simulink model "test_xeng_10_1"  (Simulink 7.2)
settings: Solver=ode45  StartTime=0.0  StopTime=400000  RelTol=1e-3
libraries: xbsIndex_r4 x840, xbsReplacements_r4 x72, casper_library x22, xps_library x3, simulink x1
(part 1 of 9)
settings Model: Creator=Jason Manley  LastModifiedBy=root
settings OptimizationCC: InitFltsAndDblsToZero=on

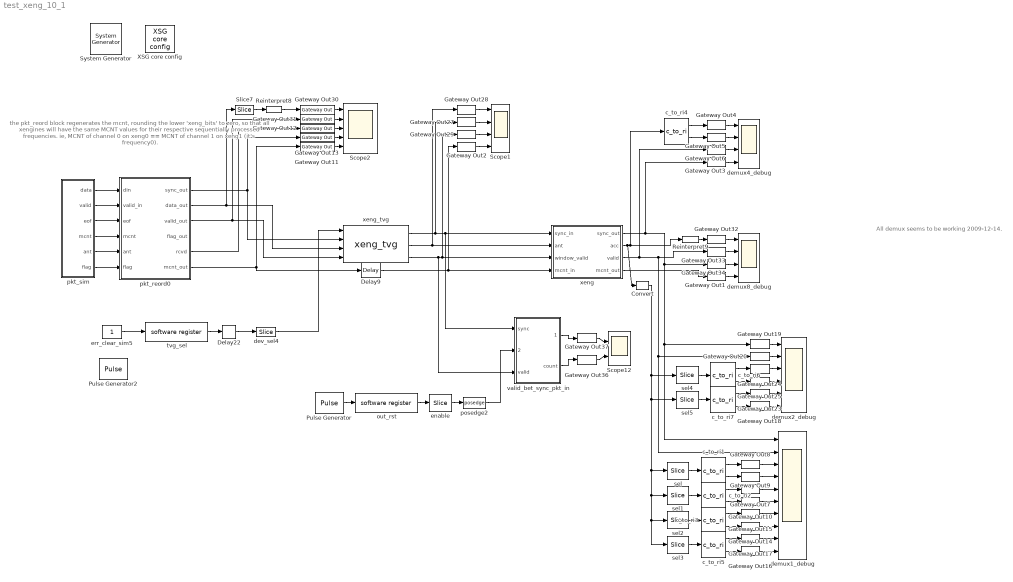
== system test_xeng_10_1 ==
  note: the pkt_reord block regenerates
      | the mcnt, rounding the lower
      | 'xeng_bits' to zero, so that all xengines
      | will have the same MCNT values for their respective
      | sequentially processed frequencies.
      | ie, MCNT of channel 0 on xeng0
      | ==
      | MCNT of channel 1 on xeng1 (it's frequency0).
  note: All demux seems to be working 2009-12-14.
  " System Generator" : xbsIndex_r4/ System Generator  Tag=genX  SystemSampleTime=-1  xilinxfamily=virtex5  part=xc5vlx110t  speed=-1  package=ff1136  synthesis_tool=XST  clock_wrapper=Clock Enables  directory=./test_vacc_pkt_10_1/sysgen  testbench=off  simulink_period=1  sysclk_period=5  dcm_input_clock_period=100  incr_netlist=off  trim_vbits=Everywhere in SubSystem  dbl_ovrd=According to Block Masks  core_generation=According to Block Masks  run_coregen=off  deprecated_control=off  eval_field=0  block_type=sysgen
      settings: block_version=10.1.3
  Convert : xbsIndex_r4/Convert  arith_type=Unsigned  n_bits=128  bin_pt=0  quantization=Truncate  overflow=Wrap  latency=0  dbl_ovrd=off  pipeline=off  block_type=convert
      settings: block_version=10.1.3
  Delay22 : xbsIndex_r4/Delay  en=off  latency=2  dbl_ovrd=off  reg_retiming=off  block_type=delay
      settings: xl_area=[0, 0, 0, 0, 0, 0, 0]
  Delay9 : xbsIndex_r4/Delay  en=off  latency=3  dbl_ovrd=off  reg_retiming=on  block_type=delay
      settings: xl_area=[0, 0, 0, 0, 0, 0, 0]
  Gateway Out{1..10,14..20,23..25,27..29,32..34,36..37} (28 alike) : xbsIndex_r4/Gateway Out  hdl_port=off  timing_constraint=None  locs_specified=off  LOCs={}  block_type=gatewayout
      settings: infoedit="Gateway out block.  Converts Xilinx fixed point inputs into ouputs of type Simulink integer, double, or fixed point.<P><P>Hardware notes:  In hardware these blocks become top level output ports or are discarded, depending on how they are configured."  xl_area=[0, 0, 0, 0, 0, 0, 0]  block_version=10.1.3
  Gateway Out{11..13,30..31} (5 alike) : xbsIndex_r4/Gateway Out  hdl_port=on  timing_constraint=None  locs_specified=off  LOCs={}  block_type=gatewayout
      settings: infoedit="Gateway out block.  Converts Xilinx fixed point inputs into ouputs of type Simulink integer, double, or fixed point.<P><P>Hardware notes:  In hardware these blocks become top level output ports or are discarded, depending on how they are configured."  xl_area=[0, 0, 0, 0, 0, 0, 0]  block_version=10.1.3
  Pulse Generator : DiscretePulseGenerator  Period=2^15  PhaseDelay=2^14
  Pulse Generator2 : DiscretePulseGenerator  Period=100000  PhaseDelay=1
  Reinterpret8 : xbsIndex_r4/Reinterpret  force_arith_type=on  arith_type="Signed  (2's comp)"  force_bin_pt=on  bin_pt=3  block_type=reinterpret
      settings: infoedit="Changes signal type without altering the binary representation.   You can changed the signal between signed and unsigned, and relocate the binary point.<P><P>Hardware notes: In hardware this block costs nothing.<P><P>Example:  Suppose the input is 6 bits wide, signed, with 2 fractional bits, and the output is forced to unsigned with 0 fractional bits.  Then an input of -2.0 (1110.00 in binary 2's complement) becomes an output of 56 (111000 in binary)."  block_version=10.1.3
  Reinterpret9 : xbsIndex_r4/Reinterpret  force_arith_type=on  arith_type="Signed  (2's comp)"  force_bin_pt=on  bin_pt=6  block_type=reinterpret
      settings: infoedit="Changes signal type without altering the binary representation.   You can changed the signal between signed and unsigned, and relocate the binary point.<P><P>Hardware notes: In hardware this block costs nothing.<P><P>Example:  Suppose the input is 6 bits wide, signed, with 2 fractional bits, and the output is forced to unsigned with 0 fractional bits.  Then an input of -2.0 (1110.00 in binary 2's complement) becomes an output of 56 (111000 in binary)."  block_version=10.1.3
  Scope1 : Scope  NumInputPorts=4
      settings: YMin=0~0~1~1460  YMax=65000~1~1~1560  SaveName=ScopeData12
  Scope12 : Scope  NumInputPorts=2
      settings: YMin=31128.7~9840  YMax=34405.3~10060  SaveName=data_into_xeng
  Scope2 : Scope  NumInputPorts=5
      settings: YMin=0~0~0~-1~344  YMax=0.9~1~1~1~360  SaveName=ScopeData18
  Slice7 : xbsIndex_r4/Slice  nbits=4  boolean_output=off  mode=Lower Bit Location + Width  bit1=0  base1=MSB of Input  bit0=0  base0=LSB of Input  dbl_ovrd=off  block_type=slice
      settings: infoedit="Extracts a given range of bits from each input sample and presents it at the output.  The output type is ordinarily unsigned with binary point at zero, but can be Boolean when the slice is one bit wide.<P><P>Hardware notes: In hardware this block costs nothing."  block_version=10.1.3
  XSG core config : xps_library/XSG core config  Tag=xps:xsg  SystemSampleTime=-1  hw_sys=iBOB  ibob_linux=off  clk_src=sys_clk  iBOB_clk_src=sys_clk  BEE2_ctrl_clk_src=sys_clk  BEE2_usr_clk_src=sys_clk  ROACH_clk_src=arb_clk  CORR_clk_src=sys_clk  gpio_clk_io_group=iBOB:sma  gpio_clk_bit_index=0  clk_rate=100  sample_period=1  synthesis_tool=XST  mpc_type=powerpc405
  c_to_ri{1..7} (7 alike) : casper_library/Misc/c_to_ri  SystemSampleTime=-1  n_bits=16  bin_pt=6
      settings: AttributesFormatString=16_6 r/i
  demux1_debug : Scope  NumInputPorts=10
      settings: YMin=-50~-15~0~-1~-5~-5~-5~-5~-5~-5  YMax=10~15~1~1~5~5~5~5~5~5  SaveName=ScopeData6
  demux2_debug : Scope  NumInputPorts=6
      settings: YMin=-50~-15~0~-1~-5~-5  YMax=10~15~1~1~5~5  SaveName=ScopeData7
  demux4_debug : Scope  NumInputPorts=4
      settings: YMin=-50~-15~0~-1  YMax=10~15~1~1
  demux8_debug : Scope  NumInputPorts=4
      settings: YMin=-10~0~-1~-1  YMax=110~1~1~1  SaveName=ScopeData20
  dev_sel4 : xbsIndex_r4/Slice  nbits=2  boolean_output=off  mode=Lower Bit Location + Width  bit1=0  base1=MSB of Input  bit0=0  base0=LSB of Input  dbl_ovrd=off  block_type=slice
      settings: infoedit="Extracts a given range of bits from each input sample and presents it at the output.  The output type is ordinarily unsigned with binary point at zero, but can be Boolean when the slice is one bit wide.<P><P>Hardware notes: In hardware this block costs nothing."  block_version=10.1.3
  enable : xbsIndex_r4/Slice  nbits=1  boolean_output=on  mode=Lower Bit Location + Width  bit1=0  base1=LSB of Input  bit0=0  base0=LSB of Input  dbl_ovrd=off  block_type=slice
      settings: infoedit="Extracts a given range of bits from each input sample and presents it at the output.  The output type is ordinarily unsigned with binary point at zero, but can be Boolean when the slice is one bit wide.<P><P>Hardware notes: In hardware this block costs nothing."  block_version=10.1.3
  err_clear_sim5 : Constant  OutDataType=sfix(16)  OutScaling=2^0
  out_rst : xps_library/software register  Tag=xps:sw_reg  SystemSampleTime=-1  io_dir=From Processor  arith_type=Unsigned  bitwidth=32  bin_pt=0  sample_period=1  gw_name=test_xeng_10_1_out_rst_user_data_out
      link override test_x_eng_nw_sim_pkt_4a_10_1_out_rst_user_data_out: arith_type=Unsigned  n_bits=32  bin_pt=0  period=1
      link override test_x_eng_sim_packet_4a_10_1_out_rst_user_data_out: arith_type=Unsigned  n_bits=32  bin_pt=0  period=1
      link override test_x_eng_sim_pkt_4a_10_1_new_out_rst_user_data_out: arith_type=Unsigned  n_bits=32  bin_pt=0  period=1
      link override test_xeng_10_1_out_rst_user_data_out: arith_type=Unsigned  n_bits=32  bin_pt=0  period=1
      link override xeng_sim_8a_out_rst_user_data_out: arith_type=Unsigned  n_bits=32  bin_pt=0  period=1
      link override xflow_sim_8a_out_rst_user_data_out: arith_type=Unsigned  n_bits=32  bin_pt=0  period=1
      link override xflow_sim_out_rst_user_data_out: arith_type=Unsigned  n_bits=32  bin_pt=0  period=1
  pkt_reord0 : Subsystem  mask{ant_bits=3, xeng_bits=3, chan_bits=7, x_int_bits=7, window_bits=3}
      mask prompts: ant_bits "Maximum Number of Antennas (2^?):"; xeng_bits "Number of Xengines in the system (2^?)"; chan_bits "Number of frequency channels in the system (2^?)"; x_int_bits "X Engine Integration Length (2^?):"; window_bits "Number of Windows to Buffer (2^?):"
      mask init:
      | sync_bits=chan_bits+x_int_bits+ant_bits-xeng_bits
      | 
      | fmtstr = sprintf('Sync period: 2^%d\nPayload Len: %i', sync_bits,2^(x_int_bits - 2));
      | set_param(gcb, 'AttributesFormatString', fmtstr);
      settings: AttributesFormatString=|
      | Sync period: 2^14
      | Payload Len: 32
  pkt_sim : Subsystem  mask{n_ants=8, n_xeng=8, xeng_int_len=128}
      mask prompts: n_ants "number of antennas in system"; n_xeng "number of x engines in system"; xeng_int_len "xeng integration length"
      mask init:
      | ants_bits = ceil(log2(n_ants));
      | xeng_bits = ceil(log2(n_xeng));
      | xeng_int_len_bits = ceil(log2(xeng_int_len));
  posedge2 : casper_library/Misc/posedge  Tag=Rising Edge Detector  SystemSampleTime=-1
  sel : xbsIndex_r4/Slice  nbits=32  boolean_output=off  mode=Lower Bit Location + Width  bit1=0  base1=LSB of Input  bit0=3*32  base0=LSB of Input  dbl_ovrd=off  block_type=slice
      settings: infoedit="Extracts a given range of bits from each input sample and presents it at the output.  The output type is ordinarily unsigned with binary point at zero, but can be Boolean when the slice is one bit wide.<P><P>Hardware notes: In hardware this block costs nothing."  block_version=10.1.3
  sel1 : xbsIndex_r4/Slice  nbits=32  boolean_output=off  mode=Lower Bit Location + Width  bit1=0  base1=LSB of Input  bit0=2*32  base0=LSB of Input  dbl_ovrd=off  block_type=slice
      settings: infoedit="Extracts a given range of bits from each input sample and presents it at the output.  The output type is ordinarily unsigned with binary point at zero, but can be Boolean when the slice is one bit wide.<P><P>Hardware notes: In hardware this block costs nothing."  block_version=10.1.3
  sel2 : xbsIndex_r4/Slice  nbits=32  boolean_output=off  mode=Lower Bit Location + Width  bit1=0  base1=LSB of Input  bit0=1*32  base0=LSB of Input  dbl_ovrd=off  block_type=slice
      settings: infoedit="Extracts a given range of bits from each input sample and presents it at the output.  The output type is ordinarily unsigned with binary point at zero, but can be Boolean when the slice is one bit wide.<P><P>Hardware notes: In hardware this block costs nothing."  block_version=10.1.3
  sel3 : xbsIndex_r4/Slice  nbits=32  boolean_output=off  mode=Lower Bit Location + Width  bit1=0  base1=LSB of Input  bit0=0*32  base0=LSB of Input  dbl_ovrd=off  block_type=slice
      settings: infoedit="Extracts a given range of bits from each input sample and presents it at the output.  The output type is ordinarily unsigned with binary point at zero, but can be Boolean when the slice is one bit wide.<P><P>Hardware notes: In hardware this block costs nothing."  block_version=10.1.3
  sel4 : xbsIndex_r4/Slice  nbits=32  boolean_output=off  mode=Lower Bit Location + Width  bit1=0  base1=LSB of Input  bit0=1*32  base0=LSB of Input  dbl_ovrd=off  block_type=slice
      settings: infoedit="Extracts a given range of bits from each input sample and presents it at the output.  The output type is ordinarily unsigned with binary point at zero, but can be Boolean when the slice is one bit wide.<P><P>Hardware notes: In hardware this block costs nothing."  block_version=10.1.3
  sel5 : xbsIndex_r4/Slice  nbits=32  boolean_output=off  mode=Lower Bit Location + Width  bit1=0  base1=LSB of Input  bit0=0*32  base0=LSB of Input  dbl_ovrd=off  block_type=slice
      settings: infoedit="Extracts a given range of bits from each input sample and presents it at the output.  The output type is ordinarily unsigned with binary point at zero, but can be Boolean when the slice is one bit wide.<P><P>Hardware notes: In hardware this block costs nothing."  block_version=10.1.3
  tvg_sel : xps_library/software register  Tag=xps:sw_reg  SystemSampleTime=-1  io_dir=From Processor  arith_type=Unsigned  bitwidth=32  bin_pt=0  sample_period=1  gw_name=test_xeng_10_1_tvg_sel_user_data_out
      link override test_x_eng_nw_sim_pkt_4a_10_1_tvg_sel_user_data_out: arith_type=Unsigned  n_bits=32  bin_pt=0  period=1
      link override test_x_eng_sim_packet_4a_10_1_tvg_sel_user_data_out: arith_type=Unsigned  n_bits=32  bin_pt=0  period=1
      link override test_x_eng_sim_pkt_4a_10_1_new_tvg_sel_user_data_out: arith_type=Unsigned  n_bits=32  bin_pt=0  period=1
      link override test_xeng_10_1_tvg_sel_user_data_out: arith_type=Unsigned  n_bits=32  bin_pt=0  period=1
      link override xeng_sim_8a_tvg_sel_user_data_out: arith_type=Unsigned  n_bits=32  bin_pt=0  period=1
      link override xflow_sim_8a_tvg_sel_user_data_out: arith_type=Unsigned  n_bits=32  bin_pt=0  period=1
      link override xflow_sim_tvg_sel_user_data_out: arith_type=Unsigned  n_bits=32  bin_pt=0  period=1
  valid_bet_sync_pkt_in : Subsystem
  xeng : Subsystem  AncestorBlock=casper_library/Correlator/xeng  mask(xeng){n_ants=8, n_bits=4, acc_len=128, demux_factor=8, add_latency=1, mult_latency=2, bram_latency=2, use_ded_mult=1, use_bram_delay=1}
      mask prompts: n_ants "Number of antennas"; n_bits "Bit-width of samples in"; acc_len "Accumulation length"; add_latency "Adder latency"; mult_latency "Multiplier latency"; bram_latency "BRAM latency"; use_ded_mult "Implementation: Multiplier type (0=slices 1=embedded 2=bram)"; use_bram_delay "Implementation: Delay type (0=SLR, 1=BRAM)"
      mask help: CASPER X engine with added internal valid data masking functionality, descramble and integral demux. Based on Aaron Parsons' and Lynn Urry's original X engine design.
      mask init:
      | xeng_init(gcb, ...
      |     'n_ants', n_ants, ...
      |     'n_bits', n_bits, ...
      |     'acc_len', acc_len, ...
      |     'demux_factor', demux_factor, ...
      |     'add_latency', add_latency, ...
      |     'mult_latency', mult_latency, ...
      |     'bram_latency', bram_latency, ...
      |     'use_ded_mult', use_ded_mult, ...
      |     'use_bram_delay', use_bram_delay);
      settings: AttributesFormatString=n_ant=8, bits=4, mult=1, bram=1
      mask StyleString: edit,edit,edit,popup(1|2|4|8),edit,edit,edit,edit,edit
  xeng_tvg : casper_library/Correlator/xeng_tvg  SystemSampleTime=-1  ant_bits=3  x_int_bits=7  sync_period=13
      link override tv0/test_xeng_10_1_xeng_tvg_tv0_user_data_out: arith_type=Unsigned  n_bits=32  bin_pt=0  period=1
      link override tv0/xeng_sim_8a_xeng_tvg_tv0_user_data_out: arith_type=Unsigned  n_bits=32  bin_pt=0  period=1
      link override tv0/xflow_sim_8a_xeng_tvg_tv0_user_data_out: arith_type=Unsigned  n_bits=32  bin_pt=0  period=1
      link override tv0/xflow_sim_xeng_tvg_tv0_user_data_out: arith_type=Unsigned  n_bits=32  bin_pt=0  period=1
      link override tv1/test_xeng_10_1_xeng_tvg_tv1_user_data_out: arith_type=Unsigned  n_bits=32  bin_pt=0  period=1
      link override tv1/xeng_sim_8a_xeng_tvg_tv1_user_data_out: arith_type=Unsigned  n_bits=32  bin_pt=0  period=1
      link override tv1/xflow_sim_8a_xeng_tvg_tv1_user_data_out: arith_type=Unsigned  n_bits=32  bin_pt=0  period=1
      link override tv1/xflow_sim_xeng_tvg_tv1_user_data_out: arith_type=Unsigned  n_bits=32  bin_pt=0  period=1
      link override tv2/test_xeng_10_1_xeng_tvg_tv2_user_data_out: arith_type=Unsigned  n_bits=32  bin_pt=0  period=1
      link override tv2/xeng_sim_8a_xeng_tvg_tv2_user_data_out: arith_type=Unsigned  n_bits=32  bin_pt=0  period=1
      link override tv2/xflow_sim_8a_xeng_tvg_tv2_user_data_out: arith_type=Unsigned  n_bits=32  bin_pt=0  period=1
      link override tv2/xflow_sim_xeng_tvg_tv2_user_data_out: arith_type=Unsigned  n_bits=32  bin_pt=0  period=1
      link override tv3/test_xeng_10_1_xeng_tvg_tv3_user_data_out: arith_type=Unsigned  n_bits=32  bin_pt=0  period=1
      link override tv3/xeng_sim_8a_xeng_tvg_tv3_user_data_out: arith_type=Unsigned  n_bits=32  bin_pt=0  period=1
      link override tv3/xflow_sim_8a_xeng_tvg_tv3_user_data_out: arith_type=Unsigned  n_bits=32  bin_pt=0  period=1
      link override tv3/xflow_sim_xeng_tvg_tv3_user_data_out: arith_type=Unsigned  n_bits=32  bin_pt=0  period=1
      link override tv4/test_xeng_10_1_xeng_tvg_tv4_user_data_out: arith_type=Unsigned  n_bits=32  bin_pt=0  period=1
      link override tv4/xeng_sim_8a_xeng_tvg_tv4_user_data_out: arith_type=Unsigned  n_bits=32  bin_pt=0  period=1
      link override tv4/xflow_sim_8a_xeng_tvg_tv4_user_data_out: arith_type=Unsigned  n_bits=32  bin_pt=0  period=1
      link override tv4/xflow_sim_xeng_tvg_tv4_user_data_out: arith_type=Unsigned  n_bits=32  bin_pt=0  period=1
      link override tv5/test_xeng_10_1_xeng_tvg_tv5_user_data_out: arith_type=Unsigned  n_bits=32  bin_pt=0  period=1
      link override tv5/xeng_sim_8a_xeng_tvg_tv5_user_data_out: arith_type=Unsigned  n_bits=32  bin_pt=0  period=1
      link override tv5/xflow_sim_8a_xeng_tvg_tv5_user_data_out: arith_type=Unsigned  n_bits=32  bin_pt=0  period=1
      link override tv5/xflow_sim_xeng_tvg_tv5_user_data_out: arith_type=Unsigned  n_bits=32  bin_pt=0  period=1
      link override tv6/test_xeng_10_1_xeng_tvg_tv6_user_data_out: arith_type=Unsigned  n_bits=32  bin_pt=0  period=1
      link override tv6/xeng_sim_8a_xeng_tvg_tv6_user_data_out: arith_type=Unsigned  n_bits=32  bin_pt=0  period=1
      link override tv6/xflow_sim_8a_xeng_tvg_tv6_user_data_out: arith_type=Unsigned  n_bits=32  bin_pt=0  period=1
      link override tv6/xflow_sim_xeng_tvg_tv6_user_data_out: arith_type=Unsigned  n_bits=32  bin_pt=0  period=1
      link override tv7/test_xeng_10_1_xeng_tvg_tv7_user_data_out: arith_type=Unsigned  n_bits=32  bin_pt=0  period=1
      link override tv7/xeng_sim_8a_xeng_tvg_tv7_user_data_out: arith_type=Unsigned  n_bits=32  bin_pt=0  period=1
      link override tv7/xflow_sim_8a_xeng_tvg_tv7_user_data_out: arith_type=Unsigned  n_bits=32  bin_pt=0  period=1
      link override tv7/xflow_sim_xeng_tvg_tv7_user_data_out: arith_type=Unsigned  n_bits=32  bin_pt=0  period=1
  wires:
  xeng_tvg/2 -> Gateway Out28/1, xeng/2(ant)
  out_rst/1 -> enable/1
  Pulse Generator/1 -> out_rst/1
  enable/1 -> posedge2/1
  posedge2/1 -> valid_bet_sync_pkt_in/2(rst_max)
  Gateway Out30/1 -> Scope2/1
  Gateway Out31/1 -> Scope2/2
  Gateway Out12/1 -> Scope2/3
  Gateway Out13/1 -> Scope2/4
  pkt_reord0/2(data_out) -> Slice7/1, xeng_tvg/3
  pkt_reord0/3(valid_out) -> Gateway Out31/1, xeng_tvg/4
  pkt_reord0/5(rcvd) -> Gateway Out12/1
  pkt_reord0/1(sync_out) -> Gateway Out13/1, xeng_tvg/2
  tvg_sel/1 -> Delay22/1
  Delay22/1 -> dev_sel4/1
  dev_sel4/1 -> xeng_tvg/1
  Gateway Out36/1 -> Scope12/2
  Gateway Out37/1 -> Scope12/1
  valid_bet_sync_pkt_in/1(max_count) -> Gateway Out37/1
  valid_bet_sync_pkt_in/2(count) -> Gateway Out36/1
  pkt_sim/6(flag) -> pkt_reord0/6(flag)
  pkt_sim/1(data) -> pkt_reord0/1(din)
  xeng_tvg/3 -> valid_bet_sync_pkt_in/3(valid), Gateway Out29/1, xeng/3(window_valid)
  xeng_tvg/1 -> Gateway Out27/1, valid_bet_sync_pkt_in/1(sync), xeng/1(sync_in)
  Gateway Out27/1 -> Scope1/2
  Gateway Out28/1 -> Scope1/1
  Gateway Out29/1 -> Scope1/3
  xeng/3(valid) -> Gateway Out6/1, Gateway Out33/1, demux1_debug/2, Gateway Out20/1
  xeng/1(sync_out) -> Gateway Out3/1, Gateway Out34/1, demux1_debug/1, Gateway Out19/1
  c_to_ri4/1 -> Gateway Out4/1
  c_to_ri4/2 -> Gateway Out5/1
  xeng/2(acc) -> c_to_ri4/1, Reinterpret9/1, Convert/1
  Gateway Out11/1 -> Scope2/5
  pkt_reord0/6(mcnt_out) -> Gateway Out11/1, Delay9/1
  Slice7/1 -> Reinterpret8/1
  Reinterpret8/1 -> Gateway Out30/1
  Gateway Out34/1 -> demux8_debug/3
  Gateway Out33/1 -> demux8_debug/2
  Gateway Out32/1 -> demux8_debug/1
  Reinterpret9/1 -> Gateway Out32/1
  pkt_sim/2(valid) -> pkt_reord0/2(valid_in)
  pkt_sim/3(eof) -> pkt_reord0/3(eof)
  pkt_sim/4(mcnt) -> pkt_reord0/4(mcnt)
  pkt_sim/5(ant) -> pkt_reord0/5(ant)
  Gateway Out1/1 -> demux8_debug/4
  xeng/4(mcnt_out) -> Gateway Out1/1
  Delay9/1 -> Gateway Out2/1, xeng/4(mcnt_in)
  Gateway Out2/1 -> Scope1/4
  err_clear_sim5/1 -> tvg_sel/1
  Gateway Out6/1 -> demux4_debug/3
  Gateway Out5/1 -> demux4_debug/2
  Gateway Out4/1 -> demux4_debug/1
  Gateway Out3/1 -> demux4_debug/4
  c_to_ri1/1 -> Gateway Out8/1
  c_to_ri1/2 -> Gateway Out9/1
  sel/1 -> c_to_ri1/1
  Gateway Out8/1 -> demux1_debug/3
  Gateway Out9/1 -> demux1_debug/4
  c_to_ri2/1 -> Gateway Out7/1
  c_to_ri2/2 -> Gateway Out10/1
  sel1/1 -> c_to_ri2/1
  c_to_ri3/1 -> Gateway Out15/1
  c_to_ri3/2 -> Gateway Out14/1
  sel2/1 -> c_to_ri3/1
  c_to_ri5/1 -> Gateway Out17/1
  c_to_ri5/2 -> Gateway Out16/1
  sel3/1 -> c_to_ri5/1
  Gateway Out7/1 -> demux1_debug/5
  Gateway Out10/1 -> demux1_debug/6
  Gateway Out15/1 -> demux1_debug/7
  Gateway Out14/1 -> demux1_debug/8
  Gateway Out17/1 -> demux1_debug/9
  Gateway Out16/1 -> demux1_debug/10
  c_to_ri6/1 -> Gateway Out24/1
  c_to_ri6/2 -> Gateway Out25/1
  sel4/1 -> c_to_ri6/1
  Gateway Out24/1 -> demux2_debug/3
  Gateway Out25/1 -> demux2_debug/4
  c_to_ri7/1 -> Gateway Out23/1
  c_to_ri7/2 -> Gateway Out18/1
  sel5/1 -> c_to_ri7/1
  Gateway Out23/1 -> demux2_debug/5
  Gateway Out18/1 -> demux2_debug/6
  Convert/1 -> sel4/1, sel/1, sel1/1, sel2/1, sel3/1, sel5/1
  Gateway Out19/1 -> demux2_debug/1
  Gateway Out20/1 -> demux2_debug/2

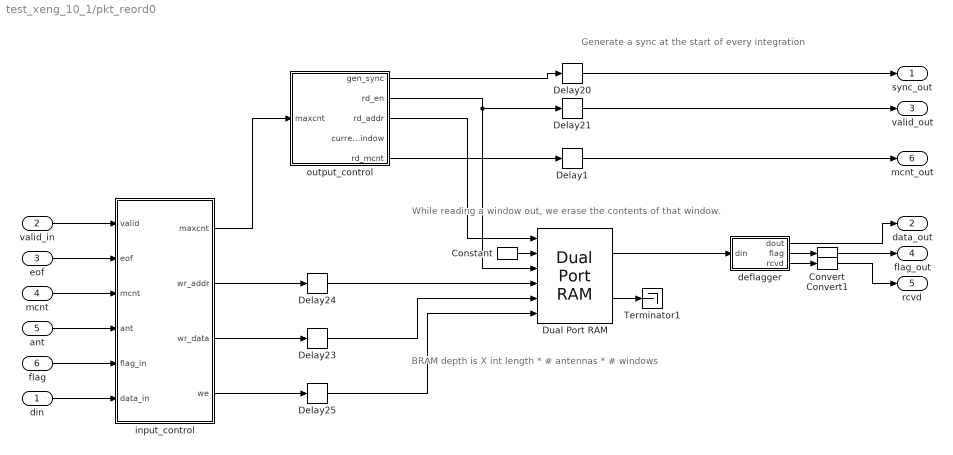
== system test_xeng_10_1/pkt_reord0 ==
  note: BRAM depth is
      | X int length * # antennas * # windows
  note: While reading a window out,
      | we erase the contents of that window.
  note: Generate a sync at the
      | start of every integration
  din : Inport  OutDataType=sfix(16)  OutScaling=2^0
  valid_in : Inport  Port=2  OutDataType=sfix(16)  OutScaling=2^0
  eof : Inport  Port=3  OutDataType=sfix(16)  OutScaling=2^0
  mcnt : Inport  Port=4  OutDataType=sfix(16)  OutScaling=2^0
  ant : Inport  Port=5  OutDataType=sfix(16)  OutScaling=2^0
  flag : Inport  Port=6  OutDataType=sfix(16)  OutScaling=2^0
  Constant : xbsIndex_r4/Constant  arith_type=Unsigned  const=0  n_bits=18  bin_pt=0  explicit_period=on  period=1  equ=P=C  opselect=C  inp2=PCIN>>17  opr=+  inp1=P  carry=CIN  dbl_ovrd=off  block_type=constant
  Convert : xbsIndex_r4/Convert  arith_type=Boolean  n_bits=16  bin_pt=14  quantization=Truncate  overflow=Wrap  latency=0  dbl_ovrd=off  pipeline=off  block_type=convert
      settings: block_version=10.1.3
  Convert1 : xbsIndex_r4/Convert  arith_type=Boolean  n_bits=16  bin_pt=14  quantization=Truncate  overflow=Wrap  latency=0  dbl_ovrd=off  pipeline=off  block_type=convert
      settings: block_version=10.1.3
  Delay1 : xbsIndex_r4/Delay  en=off  latency=3  dbl_ovrd=off  reg_retiming=on  block_type=delay
      settings: xl_area=[0, 0, 0, 0, 0, 0, 0]
  Delay20 : xbsIndex_r4/Delay  en=off  latency=3  dbl_ovrd=off  reg_retiming=on  block_type=delay
      settings: xl_area=[0, 0, 0, 0, 0, 0, 0]
  Delay21 : xbsIndex_r4/Delay  en=off  latency=3  dbl_ovrd=off  reg_retiming=on  block_type=delay
      settings: xl_area=[0, 0, 0, 0, 0, 0, 0]
  Delay23 : xbsIndex_r4/Delay  en=off  latency=2  dbl_ovrd=off  reg_retiming=on  block_type=delay
      settings: xl_area=[0, 0, 0, 0, 0, 0, 0]
  Delay24 : xbsIndex_r4/Delay  en=off  latency=2  dbl_ovrd=off  reg_retiming=on  block_type=delay
      settings: xl_area=[0, 0, 0, 0, 0, 0, 0]
  Delay25 : xbsIndex_r4/Delay  en=off  latency=2  dbl_ovrd=off  reg_retiming=on  block_type=delay
      settings: xl_area=[0, 0, 0, 0, 0, 0, 0]
  Dual Port RAM : xbsIndex_r4/Dual Port RAM  depth=2^x_int_bits * 2^ant_bits * 2^window_bits  initVector=1  distributed_mem=Block RAM  init_a=0  init_b=0  rst_a=off  rst_b=off  en_a=off  en_b=off  latency=3  write_mode_A=Read Before Write  write_mode_B=Read Before Write  dbl_ovrd=off  optimize=Area  use_rpm=off  block_type=dpram
      settings: xl_area=[0, 0, 0, 0, 0, 0, 0]  block_version=10.1.3
  Terminator1 : Terminator
  deflagger : Subsystem
  input_control : Subsystem
  output_control : Subsystem
  sync_out : Outport  OutDataType=sfix(16)  OutScaling=2^0
  data_out : Outport  Port=2  OutDataType=sfix(16)  OutScaling=2^0
  valid_out : Outport  Port=3  OutDataType=sfix(16)  OutScaling=2^0
  flag_out : Outport  Port=4  OutDataType=sfix(16)  OutScaling=2^0
  rcvd : Outport  Port=5  OutDataType=sfix(16)  OutScaling=2^0
  mcnt_out : Outport  Port=6  OutDataType=sfix(16)  OutScaling=2^0
  wires:
  input_control/4(we) -> Delay25/1
  input_control/2(wr_addr) -> Delay24/1
  output_control/2(rd_en) -> Dual Port RAM/3, Delay21/1
  output_control/3(rd_addr) -> Dual Port RAM/1
  Constant/1 -> Dual Port RAM/2
  deflagger/3(rcvd) -> Convert1/1
  deflagger/2(flag) -> Convert/1
  deflagger/1(dout) -> data_out/1
  Delay21/1 -> valid_out/1
  valid_in/1 -> input_control/1(valid)
  eof/1 -> input_control/2(eof)
  ant/1 -> input_control/4(ant)
  mcnt/1 -> input_control/3(mcnt)
  Delay20/1 -> sync_out/1
  Dual Port RAM/2 -> Terminator1/1
  Dual Port RAM/1 -> deflagger/1(din)
  output_control/1(gen_sync) -> Delay20/1
  input_control/3(wr_data) -> Delay23/1
  din/1 -> input_control/6(data_in)
  flag/1 -> input_control/5(flag_in)
  input_control/1(maxcnt) -> output_control/1(maxcnt)
  Delay24/1 -> Dual Port RAM/4
  Delay23/1 -> Dual Port RAM/5
  Delay25/1 -> Dual Port RAM/6
  output_control/5(rd_mcnt) -> Delay1/1
  Delay1/1 -> mcnt_out/1
  Convert/1 -> flag_out/1
  Convert1/1 -> rcvd/1

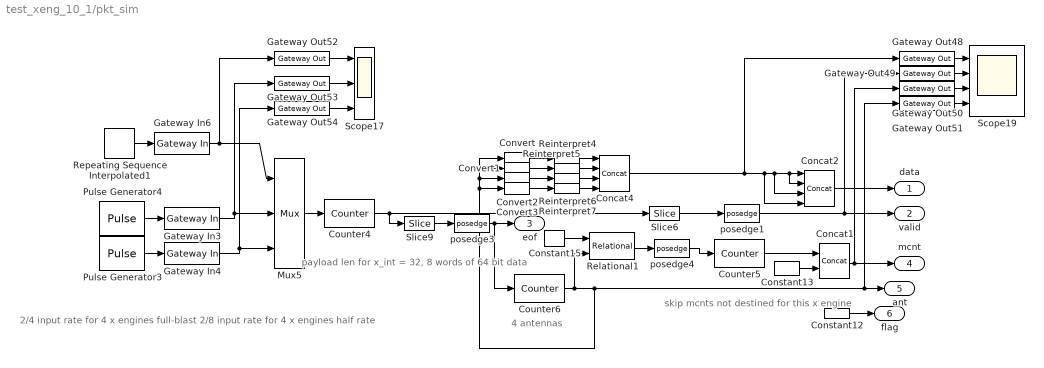
== system test_xeng_10_1/pkt_sim ==
  note: 2/4 input rate for 4 x engines full-blast
      | 2/8 input rate for 4 x engines half rate
  note: 4 antennas
  note: skip mcnts not destined
      | for this x engine
  note: payload len
      | for x_int = 32,
      | 8 words of 64 bit data
  Concat1 : xbsIndex_r4/Concat  num_inputs=2  dbl_ovrd=off  block_type=concat
      settings: block_version=10.1.3
  Concat2 : xbsIndex_r4/Concat  num_inputs=4  dbl_ovrd=off  block_type=concat
      settings: block_version=10.1.3
  Concat4 : xbsIndex_r4/Concat  num_inputs=4  dbl_ovrd=off  block_type=concat
      settings: block_version=10.1.3
  Constant12 : xbsIndex_r4/Constant  arith_type=Unsigned  const=0  n_bits=1  bin_pt=0  explicit_period=on  period=1  equ=P=C  opselect=C  inp2=PCIN>>17  opr=+  inp1=P  carry=CIN  dbl_ovrd=off  block_type=constant
  Constant13 : xbsIndex_r4/Constant  arith_type=Unsigned  const=0  n_bits=ants_bits  bin_pt=0  explicit_period=on  period=1  equ=P=C  opselect=C  inp2=PCIN>>17  opr=+  inp1=P  carry=CIN  dbl_ovrd=off  block_type=constant
  Constant15 : xbsIndex_r4/Constant  arith_type=Unsigned  const=0  n_bits=ants_bits  bin_pt=0  explicit_period=on  period=1  equ=P=C  opselect=C  inp2=PCIN>>17  opr=+  inp1=P  carry=CIN  dbl_ovrd=off  block_type=constant
  Convert{,1..3} (4 alike) : xbsIndex_r4/Convert  arith_type="Signed  (2's comp)"  n_bits=4  bin_pt=0  quantization=Truncate  overflow=Saturate  latency=0  dbl_ovrd=off  pipeline=off  block_type=convert
      settings: block_version=10.1.3
  Counter4 : xbsIndex_r4/Counter  cnt_type=Free Running  cnt_to=32  operation=Up  start_count=0  cnt_by_val=1  arith_type=Unsigned  n_bits=32  bin_pt=0  load_pin=off  rst=off  en=on  explicit_period=off  period=1  dbl_ovrd=off  use_behavioral_HDL=off  implementation=Fabric  use_rpm=on  block_type=counter
      settings: xl_area=[0, 0, 0, 0, 0, 0, 0]
  Counter5 : xbsIndex_r4/Counter  cnt_type=Free Running  cnt_to=Inf  operation=Up  start_count=0  cnt_by_val=1  arith_type=Unsigned  n_bits=48-ants_bits  bin_pt=0  load_pin=off  rst=off  en=on  explicit_period=off  period=1  dbl_ovrd=off  use_behavioral_HDL=off  implementation=Fabric  use_rpm=on  block_type=counter
      settings: xl_area=[0, 0, 0, 0, 0, 0, 0]
  Counter6 : xbsIndex_r4/Counter  cnt_type=Free Running  cnt_to=Inf  operation=Up  start_count=0  cnt_by_val=1  arith_type=Unsigned  n_bits=ants_bits  bin_pt=0  load_pin=off  rst=off  en=on  explicit_period=off  period=1  dbl_ovrd=off  use_behavioral_HDL=off  implementation=Fabric  use_rpm=on  block_type=counter
      settings: xl_area=[0, 0, 0, 0, 0, 0, 0]
  Gateway In3 : xbsIndex_r4/Gateway In  arith_type=Boolean  n_bits=8  bin_pt=6  quantization=Truncate  overflow=Wrap  period=1  dbl_ovrd=off  timing_constraint=None  locs_specified=off  LOCs={}  hdl_port=on  block_type=gatewayin
      settings: infoedit="Gateway in block.  Converts inputs of type Simulink integer, double and fixed point to  Xilinx fixed point type.<P><P>Hardware notes:  In hardware these blocks become top level input ports."  xl_area=[0, 0, 0, 0, 0, 0, 0]  block_version=10.1.3
  Gateway In4 : xbsIndex_r4/Gateway In  arith_type=Boolean  n_bits=8  bin_pt=6  quantization=Truncate  overflow=Wrap  period=1  dbl_ovrd=off  timing_constraint=None  locs_specified=off  LOCs={}  hdl_port=on  block_type=gatewayin
      settings: infoedit="Gateway in block.  Converts inputs of type Simulink integer, double and fixed point to  Xilinx fixed point type.<P><P>Hardware notes:  In hardware these blocks become top level input ports."  xl_area=[0, 0, 0, 0, 0, 0, 0]  block_version=10.1.3
  Gateway In6 : xbsIndex_r4/Gateway In  arith_type=Unsigned  n_bits=1  bin_pt=0  quantization=Truncate  overflow=Wrap  period=1  dbl_ovrd=off  timing_constraint=None  locs_specified=off  LOCs={}  hdl_port=on  block_type=gatewayin
      settings: infoedit="Gateway in block.  Converts inputs of type Simulink integer, double and fixed point to  Xilinx fixed point type.<P><P>Hardware notes:  In hardware these blocks become top level input ports."  xl_area=[0, 0, 0, 0, 0, 0, 0]  block_version=10.1.3
  Gateway Out{48..54} (7 alike) : xbsIndex_r4/Gateway Out  hdl_port=on  timing_constraint=None  locs_specified=off  LOCs={}  block_type=gatewayout
      settings: infoedit="Gateway out block.  Converts Xilinx fixed point inputs into ouputs of type Simulink integer, double, or fixed point.<P><P>Hardware notes:  In hardware these blocks become top level output ports or are discarded, depending on how they are configured."  xl_area=[0, 0, 0, 0, 0, 0, 0]  block_version=10.1.3
  Mux5 : xbsIndex_r4/Mux  inputs=2  en=off  latency=0  precision=Full  arith_type="Signed  (2's comp)"  n_bits=8  bin_pt=2  quantization=Truncate  overflow=Wrap  dbl_ovrd=off  block_type=mux
      settings: xl_area=[0, 0, 0, 0, 0, 0, 0]
  Pulse Generator3 : DiscretePulseGenerator  Period=4  PulseWidth=2
  Pulse Generator4 : DiscretePulseGenerator  PulseWidth=2
  Reinterpret{4..7} (4 alike) : xbsIndex_r4/Reinterpret  force_arith_type=on  arith_type=Unsigned  force_bin_pt=on  bin_pt=0  block_type=reinterpret
      settings: infoedit="Changes signal type without altering the binary representation.   You can changed the signal between signed and unsigned, and relocate the binary point.<P><P>Hardware notes: In hardware this block costs nothing.<P><P>Example:  Suppose the input is 6 bits wide, signed, with 2 fractional bits, and the output is forced to unsigned with 0 fractional bits.  Then an input of -2.0 (1110.00 in binary 2's complement) becomes an output of 56 (111000 in binary)."  block_version=10.1.3
  Relational1 : xbsIndex_r4/Relational  mode=a=b  en=off  latency=1  dbl_ovrd=off  block_type=relational
      settings: xl_area=[0, 0, 0, 0, 0, 0, 0]  block_version=10.1.3
  Repeating Sequence Interpolated1 : simulink/Sources/Repeating Sequence Interpolated  SystemSampleTime=-1  OutValues=[0 1]  TimeValues=[40000 200000]  LookUpMeth=Use Input Above  tsamp=1  OutMin=[]  OutMax=[]  OutDataTypeStr=float('double')  OutputDataTypeScalingMode=Specify via dialog  OutDataType=float('double')  OutScaling=2^-10
  Scope17 : Scope  NumInputPorts=3
      settings: YMin=-1~0~0  YMax=1~1~1  SaveName=ScopeData16
  Scope19 : Scope  NumInputPorts=4
      settings: YMin=0~0~28~0  YMax=1~1~40~3  SaveName=ScopeData17
  Slice6 : xbsIndex_r4/Slice  nbits=1  boolean_output=on  mode=Lower Bit Location + Width  bit1=0  base1=MSB of Input  bit0=0  base0=LSB of Input  dbl_ovrd=off  block_type=slice
      settings: infoedit="Extracts a given range of bits from each input sample and presents it at the output.  The output type is ordinarily unsigned with binary point at zero, but can be Boolean when the slice is one bit wide.<P><P>Hardware notes: In hardware this block costs nothing."  block_version=10.1.3
  Slice9 : xbsIndex_r4/Slice  nbits=1  boolean_output=on  mode=Lower Bit Location + Width  bit1=0  base1=MSB of Input  bit0=xeng_int_len_bits-1  base0=LSB of Input  dbl_ovrd=off  block_type=slice
      settings: infoedit="Extracts a given range of bits from each input sample and presents it at the output.  The output type is ordinarily unsigned with binary point at zero, but can be Boolean when the slice is one bit wide.<P><P>Hardware notes: In hardware this block costs nothing."  block_version=10.1.3
  posedge1 : casper_library/Misc/posedge  Tag=Rising Edge Detector  SystemSampleTime=-1
  posedge3 : casper_library/Misc/posedge  Tag=Rising Edge Detector  SystemSampleTime=-1
  posedge4 : casper_library/Misc/posedge  Tag=Rising Edge Detector  SystemSampleTime=-1
  data : Outport
  valid : Outport  Port=2
  eof : Outport  Port=3
  mcnt : Outport  Port=4
  ant : Outport  Port=5
  flag : Outport  Port=6
  wires:
  Gateway Out48/1 -> Scope19/1
  Gateway Out49/1 -> Scope19/2
  Gateway Out50/1 -> Scope19/3
  Gateway Out51/1 -> Scope19/4
  Constant13/1 -> Concat1/2
  Concat1/1 -> Gateway Out50/1, mcnt/1
  Counter5/1 -> Concat1/1
  Counter6/1 -> Relational1/2, Gateway Out51/1, ant/1, Convert1/1, Convert/1, Convert2/1, Convert3/1
  Relational1/1 -> posedge4/1
  Constant15/1 -> Relational1/1
  Slice6/1 -> posedge1/1
  Counter4/1 -> Slice9/1, Slice6/1
  Slice9/1 -> posedge3/1
  posedge3/1 -> Counter6/1, eof/1
  posedge4/1 -> Counter5/1
  Pulse Generator3/1 -> Gateway In4/1
  Concat4/1 -> Concat2/4, Concat2/3, Concat2/1, Concat2/2, Gateway Out48/1
  Pulse Generator4/1 -> Gateway In3/1
  Mux5/1 -> Counter4/1
  Gateway In3/1 -> Gateway Out53/1, Mux5/2
  Gateway In4/1 -> Gateway Out54/1, Mux5/3
  Gateway In6/1 -> Mux5/1, Gateway Out52/1
  Repeating Sequence Interpolated1/1 -> Gateway In6/1
  Gateway Out52/1 -> Scope17/1
  Gateway Out53/1 -> Scope17/2
  Gateway Out54/1 -> Scope17/3
  posedge1/1 -> Gateway Out49/1, valid/1
  Convert/1 -> Reinterpret4/1
  Convert1/1 -> Reinterpret5/1
  Convert2/1 -> Reinterpret6/1
  Convert3/1 -> Reinterpret7/1
  Reinterpret4/1 -> Concat4/1
  Reinterpret6/1 -> Concat4/3
  Reinterpret7/1 -> Concat4/4
  Reinterpret5/1 -> Concat4/2
  Concat2/1 -> data/1
  Constant12/1 -> flag/1

== system test_xeng_10_1/valid_bet_sync_pkt_in ==
  sync : Inport  OutDataType=sfix(16)  OutScaling=2^0
  rst_max : Inport  Port=2  OutDataType=sfix(16)  OutScaling=2^0
  valid : Inport  Port=3  OutDataType=sfix(16)  OutScaling=2^0
  Delay14 : xbsIndex_r4/Delay  en=off  latency=1  dbl_ovrd=off  reg_retiming=on  block_type=delay
      settings: xl_area=[0, 0, 0, 0, 0, 0, 0]
  Register3 : xbsIndex_r4/Register  init=0  rst=on  en=on  dbl_ovrd=off  block_type=register
      settings: xl_area=[0, 0, 0, 0, 0, 0, 0]
  Relational5 : xbsIndex_r4/Relational  mode=a>=b  en=off  latency=1  dbl_ovrd=off  block_type=relational
      settings: xl_area=[0, 0, 0, 0, 0, 0, 0]  block_version=10.1.3
  valid_cntr : xbsIndex_r4/Counter  cnt_type=Count Limited  cnt_to=Inf  operation=Up  start_count=0  cnt_by_val=1  arith_type="Signed  (2's comp)"  n_bits=32  bin_pt=0  load_pin=off  rst=on  en=on  explicit_period=on  period=1  dbl_ovrd=off  use_behavioral_HDL=off  implementation=Fabric  use_rpm=on  block_type=counter
      settings: xl_area=[0, 0, 0, 0, 0, 0, 0]
  max_count : Outport  OutDataType=sfix(16)  OutScaling=2^0
  count : Outport  Port=2  OutDataType=sfix(16)  OutScaling=2^0
  wires:
  Delay14/1 -> Register3/1
  Relational5/1 -> Register3/3
  Register3/1 -> Relational5/2, max_count/1
  valid_cntr/1 -> Relational5/1, Delay14/1, count/1
  sync/1 -> valid_cntr/1
  rst_max/1 -> Register3/2
  valid/1 -> valid_cntr/2

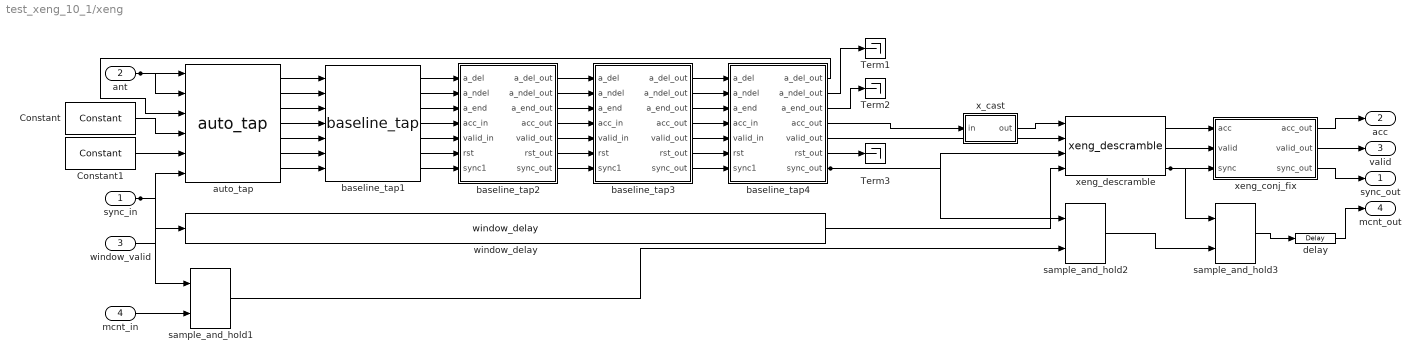
== system test_xeng_10_1/xeng ==
  sync_in : Inport
  ant : Inport  Port=2
  window_valid : Inport  Port=3
  mcnt_in : Inport  Port=4  OutDataType=sfix(16)  OutScaling=2^0
  Constant : xbsIndex_r4/Constant  arith_type=Unsigned  const=0  n_bits=128  bin_pt=14  explicit_period=off  period=1  equ=P=C  opselect=C  inp2=PCIN>>17  opr=+  inp1=P  carry=CIN  dbl_ovrd=off  block_type=constant
  Constant1 : xbsIndex_r4/Constant  arith_type=Boolean  const=0  n_bits=1  bin_pt=14  explicit_period=off  period=1  equ=P=C  opselect=C  inp2=PCIN>>17  opr=+  inp1=P  carry=CIN  dbl_ovrd=off  block_type=constant
  Term1 : Terminator
  Term2 : Terminator
  Term3 : Terminator
  auto_tap : casper_library/Correlator/auto_tap  SystemSampleTime=-1  n_ants=8  n_bits=4  acc_len=128  add_latency=1  mult_latency=2  bram_latency=2  use_ded_mult=1  use_bram_delay=1
      settings: AttributesFormatString=mult=1
  baseline_tap1 : casper_library/Correlator/baseline_tap  SystemSampleTime=-1  n_ants=8  ant_sep=1  n_bits=4  acc_len=128  add_latency=1  mult_latency=2  bram_latency=2  use_ded_mult=1  use_bram_delay=1
      settings: AttributesFormatString=ant_sep=1, mult=1, bram=1
  baseline_tap2 : Subsystem  AncestorBlock=casper_library/Correlator/baseline_tap  mask(baseline_tap){n_ants=8, ant_sep=2, n_bits=4, acc_len=128, add_latency=1, mult_latency=2, bram_latency=2, use_ded_mult=1, use_bram_delay=1}
      mask prompts: n_ants "Number of antennas"; ant_sep "Antenna Seperation"; n_bits "number of input bits (per complex component)"; acc_len "accumulation length"; add_latency "Adder latency"; mult_latency "Multiplier latency"; bram_latency "BRAM latency"; use_ded_mult "Multiplier Type (0=slices 1=embedded 2=bram)"; use_bram_delay "Use BRAM delays"
      mask init:
      | fix_pnt_pos = (n_bits-1)*2;
      | bit_growth = ceil(log2(acc_len));
      | ant_bits = ceil(log2(n_ants));
      | n_bits_out = (2*n_bits + 1 + bit_growth);
      | 
      | baseline_tap_init(gcb, ...
      |     'ant_sep', ant_sep, ...
      |     'use_ded_mult', use_ded_mult, ...
      |     'use_bram_delay', use_bram_delay);
      settings: AttributesFormatString=ant_sep=2, mult=1, bram=1
  baseline_tap3 : Subsystem  AncestorBlock=casper_library/Correlator/baseline_tap  mask(baseline_tap){n_ants=8, ant_sep=3, n_bits=4, acc_len=128, add_latency=1, mult_latency=2, bram_latency=2, use_ded_mult=1, use_bram_delay=1}
      mask prompts: n_ants "Number of antennas"; ant_sep "Antenna Seperation"; n_bits "number of input bits (per complex component)"; acc_len "accumulation length"; add_latency "Adder latency"; mult_latency "Multiplier latency"; bram_latency "BRAM latency"; use_ded_mult "Multiplier Type (0=slices 1=embedded 2=bram)"; use_bram_delay "Use BRAM delays"
      mask init: same as test_xeng_10_1/xeng/baseline_tap2
      settings: AttributesFormatString=ant_sep=3, mult=1, bram=1
  baseline_tap4 : Subsystem  AncestorBlock=casper_library/Correlator/baseline_tap  mask(baseline_tap){n_ants=8, ant_sep=4, n_bits=4, acc_len=128, add_latency=1, mult_latency=2, bram_latency=2, use_ded_mult=1, use_bram_delay=1}
      mask prompts: n_ants "Number of antennas"; ant_sep "Antenna Seperation"; n_bits "number of input bits (per complex component)"; acc_len "accumulation length"; add_latency "Adder latency"; mult_latency "Multiplier latency"; bram_latency "BRAM latency"; use_ded_mult "Multiplier Type (0=slices 1=embedded 2=bram)"; use_bram_delay "Use BRAM delays"
      mask init: same as test_xeng_10_1/xeng/baseline_tap2
      settings: AttributesFormatString=ant_sep=4, mult=1, bram=1
  delay : xbsIndex_r4/Delay  en=off  latency=1  dbl_ovrd=off  reg_retiming=on  block_type=delay
      settings: block_version=11.4
  sample_and_hold1 : casper_library/Misc/sample_and_hold  SystemSampleTime=-1  period=1024
  sample_and_hold2 : casper_library/Misc/sample_and_hold  SystemSampleTime=-1  period=1024
  sample_and_hold3 : casper_library/Misc/sample_and_hold  SystemSampleTime=-1  period=1024
  window_delay : casper_library/Delays/window_delay  SystemSampleTime=-1  delay=137
  x_cast : Subsystem  AncestorBlock=casper_library/Correlator/x_cast  mask{n_bits_in=16, n_bits_out=16, fix_pnt_pos=6, demux_factor=8}
      mask prompts: n_bits_in "Number of bits (input)"; n_bits_out "Number of bits (output)"; fix_pnt_pos "Fixed point position"; demux_factor "Demux Factor"
      mask init:
      | switch (demux_factor)
      |     case (8)
      |         bit_offsets=[0 1 2 3 4 5 6 7];
      |     case (4) 
      |         bit_offsets=[4 5 6 7 0 1 2 3];  
      |     case (2) 
      |         bit_offsets=[6 7 4 5 2 3 0 1];  
      |     case (1) 
      |         bit_offsets=[7 6 5 4 3 2 1 0];  
      | end
  xeng_conj_fix : Subsystem  AncestorBlock=casper_library/Correlator/xeng_conj_fix  mask(xeng_conj_fix){n_ants=8, n_bits_in=16, demux_factor=8}
      mask prompts: n_ants "Number of Antennas"; n_bits_in "Input Bitwidth (complex, bit width per component)"; demux_factor "Demux factor"
      mask help:
      | This block corrects the "lower triangle" of the X engine's output so that products are conjugated according to the astronomy convention of
      | lower_antenna_index * conj(higher_antenna_index).
      |
      | It expects demuxed input. Ie the ACC line contains a single complex number per clock.
      mask init:
      | xeng_conj_fix_init(gcb, 'n_ants', n_ants,...
      |     'n_bits_in',n_bits_in,...
      |     'demux_factor',demux_factor);
      | 
      | fmtstr = sprintf('num_ants=%d',n_ants);
      | set_param(gcb, 'AttributesFormatString', fmtstr);
      settings: AttributesFormatString=num_ants=8
  xeng_descramble : casper_library/Correlator/xeng_descramble  SystemSampleTime=-1  num_ants=8  n_bits_in=128  demux_factor=8  acc_len=128
      settings: AttributesFormatString=num_ants=8
  sync_out : Outport
  acc : Outport  Port=2
  valid : Outport  Port=3
  mcnt_out : Outport  Port=4
  wires:
  xeng_descramble/1 -> xeng_conj_fix/1(acc)
  xeng_descramble/2 -> xeng_conj_fix/2(valid)
  xeng_descramble/3 -> xeng_conj_fix/3(sync), sample_and_hold3/1
  x_cast/1(out) -> xeng_descramble/1
  baseline_tap4/5(valid_out) -> xeng_descramble/2
  baseline_tap4/7(sync_out) -> xeng_descramble/3, sample_and_hold2/1
  window_delay/1 -> xeng_descramble/4
  ant/1 -> auto_tap/1, auto_tap/2
  Constant/1 -> auto_tap/4
  Constant1/1 -> auto_tap/5
  sync_in/1 -> auto_tap/6, sample_and_hold1/1
  window_valid/1 -> window_delay/1
  xeng_conj_fix/3(sync_out) -> sync_out/1
  xeng_conj_fix/1(acc_out) -> acc/1
  xeng_conj_fix/2(valid_out) -> valid/1
  mcnt_in/1 -> sample_and_hold1/2
  sample_and_hold1/1 -> sample_and_hold2/2
  sample_and_hold2/1 -> sample_and_hold3/2
  sample_and_hold3/1 -> delay/1
  delay/1 -> mcnt_out/1
  auto_tap/1 -> baseline_tap1/1
  auto_tap/2 -> baseline_tap1/2
  auto_tap/3 -> baseline_tap1/3
  auto_tap/4 -> baseline_tap1/4
  auto_tap/5 -> baseline_tap1/5
  auto_tap/6 -> baseline_tap1/6
  auto_tap/7 -> baseline_tap1/7
  baseline_tap1/1 -> baseline_tap2/1(a_del)
  baseline_tap1/2 -> baseline_tap2/2(a_ndel)
  baseline_tap1/3 -> baseline_tap2/3(a_end)
  baseline_tap1/4 -> baseline_tap2/4(acc_in)
  baseline_tap1/5 -> baseline_tap2/5(valid_in)
  baseline_tap1/6 -> baseline_tap2/6(rst)
  baseline_tap1/7 -> baseline_tap2/7(sync1)
  baseline_tap2/1(a_del_out) -> baseline_tap3/1(a_del)
  baseline_tap2/2(a_ndel_out) -> baseline_tap3/2(a_ndel)
  baseline_tap2/3(a_end_out) -> baseline_tap3/3(a_end)
  baseline_tap2/4(acc_out) -> baseline_tap3/4(acc_in)
  baseline_tap2/5(valid_out) -> baseline_tap3/5(valid_in)
  baseline_tap2/6(rst_out) -> baseline_tap3/6(rst)
  baseline_tap2/7(sync_out) -> baseline_tap3/7(sync1)
  baseline_tap3/1(a_del_out) -> baseline_tap4/1(a_del)
  baseline_tap3/2(a_ndel_out) -> baseline_tap4/2(a_ndel)
  baseline_tap3/3(a_end_out) -> baseline_tap4/3(a_end)
  baseline_tap3/4(acc_out) -> baseline_tap4/4(acc_in)
  baseline_tap3/5(valid_out) -> baseline_tap4/5(valid_in)
  baseline_tap3/6(rst_out) -> baseline_tap4/6(rst)
  baseline_tap3/7(sync_out) -> baseline_tap4/7(sync1)
  baseline_tap4/1(a_del_out) -> auto_tap/3
  baseline_tap4/2(a_ndel_out) -> Term1/1
  baseline_tap4/3(a_end_out) -> Term2/1
  baseline_tap4/4(acc_out) -> x_cast/1(in)
  baseline_tap4/6(rst_out) -> Term3/1

== system test_xeng_10_1/pkt_reord0/deflagger ==
  din : Inport  OutDataType=sfix(16)  OutScaling=2^0
  Slice1 : xbsIndex_r4/Slice  nbits=16  boolean_output=off  mode=Lower Bit Location + Width  bit1=0  base1=MSB of Input  bit0=0  base0=LSB of Input  dbl_ovrd=off  block_type=slice
      settings: infoedit="Extracts a given range of bits from each input sample and presents it at the output.  The output type is ordinarily unsigned with binary point at zero, but can be Boolean when the slice is one bit wide.<P><P>Hardware notes: In hardware this block costs nothing."  block_version=10.1.3
  Slice2 : xbsIndex_r4/Slice  nbits=1  boolean_output=off  mode=Upper Bit Location + Width  bit1=-1  base1=MSB of Input  bit0=0  base0=LSB of Input  dbl_ovrd=off  block_type=slice
      settings: infoedit="Extracts a given range of bits from each input sample and presents it at the output.  The output type is ordinarily unsigned with binary point at zero, but can be Boolean when the slice is one bit wide.<P><P>Hardware notes: In hardware this block costs nothing."  block_version=10.1.3
  Slice3 : xbsIndex_r4/Slice  nbits=1  boolean_output=off  mode=Upper Bit Location + Width  bit1=0  base1=MSB of Input  bit0=0  base0=LSB of Input  dbl_ovrd=off  block_type=slice
      settings: infoedit="Extracts a given range of bits from each input sample and presents it at the output.  The output type is ordinarily unsigned with binary point at zero, but can be Boolean when the slice is one bit wide.<P><P>Hardware notes: In hardware this block costs nothing."  block_version=10.1.3
  dout : Outport  OutDataType=sfix(16)  OutScaling=2^0
  flag : Outport  Port=2  OutDataType=sfix(16)  OutScaling=2^0
  rcvd : Outport  Port=3  OutDataType=sfix(16)  OutScaling=2^0
  wires:
  Slice1/1 -> dout/1
  Slice3/1 -> rcvd/1
  Slice2/1 -> flag/1
  din/1 -> Slice3/1, Slice2/1, Slice1/1
